simulink model "karamy"  (R2016b)
settings: Solver=ode23s  StartTime=0.0  StopTime=10  RelTol=.01
InitFcn:
  | init
values from neighbouring files (symbols this model uses):
  etta0 = x(3)    [KARAMY2.m]    (also in system10.mat = 0.574023203436; system20.mat = 0.293427975482; system30.mat = 0.568096136445)
  Ksm0 = x(1)    [KARAMY2.m]    (also in system10.mat = 0.523640532645; system20.mat = 0.612490346894; system30.mat = 0.775379405953)
settings Model: Creator=Mojtaba  LastModifiedBy=Mojtaba
settings SolverCC: ShapePreserveControl=EnableAll

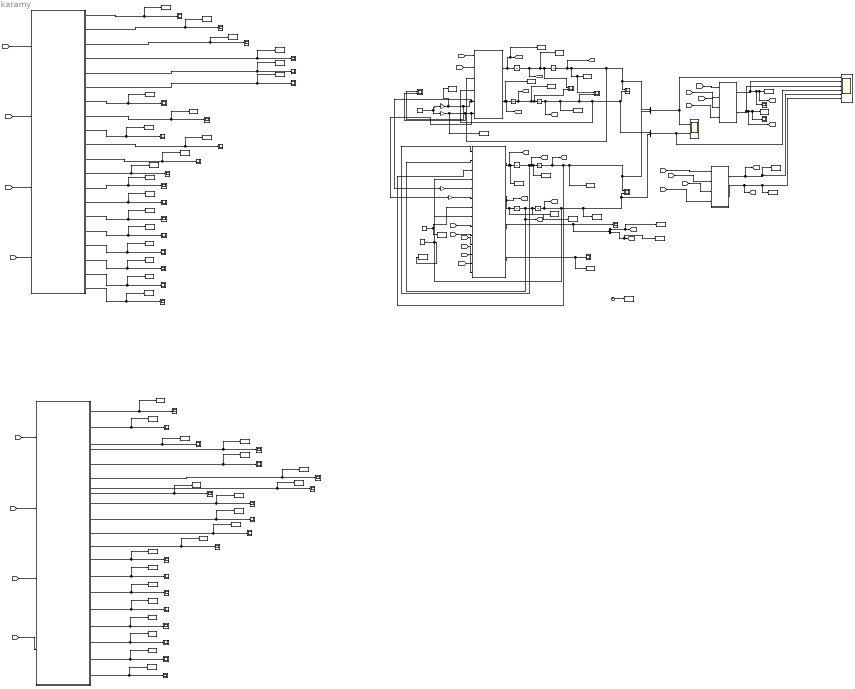
== system karamy ==
  Clock : Clock
  Constant : Constant  Value=Ksm0
  Constant1 : Constant  Value=etta0
  Demux : Demux  Outputs=2
  Dis : SignalGenerator  Amplitude=.1  Units=rad/sec
  Gain{,1..3} (4 alike) : Gain
  Integrator10 : Integrator  InitialCondition=.6
  Integrator11 : Integrator  InitialCondition=.1
  Integrator{8..9,12..13} (4 alike) : Integrator
  Integrator14 : Integrator  InitialCondition=.6
  Integrator15 : Integrator  InitialCondition=.1
  "Muscle1 " : MATLAB Function  TreatAsAtomicUnit=on
  Muscle2 : MATLAB Function  TreatAsAtomicUnit=on
  Mux5 : Mux  Inputs=2
  Mux6 : Mux  Inputs=2
  Subsystem10 : Subsystem
  Subsystem13 : Subsystem
  To Workspace : ToWorkspace  VariableName=u1  SampleTime=-1
  To Workspace1 : ToWorkspace  VariableName=ddqO2  SampleTime=-1
  To Workspace10 : ToWorkspace  VariableName=dqO1  SampleTime=-1
  To Workspace11 : ToWorkspace  VariableName=ddqO1  SampleTime=-1
  To Workspace12 : ToWorkspace  VariableName=qC1  SampleTime=-1
  To Workspace13 : ToWorkspace  VariableName=ddqC2  SampleTime=-1
  To Workspace14 : ToWorkspace  VariableName=ddxR2  SampleTime=-1
  To Workspace15 : ToWorkspace  VariableName=ddxL2  SampleTime=-1
  To Workspace16 : ToWorkspace  VariableName=ddxR1  SampleTime=-1
  To Workspace17 : ToWorkspace  VariableName=Ksm  SampleTime=-1
  To Workspace18 : ToWorkspace  VariableName=dis1  SampleTime=-1
  To Workspace19 : ToWorkspace  VariableName=dqO2  SampleTime=-1
  To Workspace2 : ToWorkspace  VariableName=time  SampleTime=-1
  To Workspace20 : ToWorkspace  VariableName=qO2  SampleTime=-1
  To Workspace21 : ToWorkspace  VariableName=dqC2  SampleTime=-1
  To Workspace22 : ToWorkspace  VariableName=ddxL1  SampleTime=-1
  To Workspace25 : ToWorkspace  VariableName=u2  SampleTime=-1
  To Workspace26 : ToWorkspace  VariableName=qO1  SampleTime=-1
  To Workspace27 : ToWorkspace  VariableName=dqC1  SampleTime=-1
  To Workspace28 : ToWorkspace  VariableName=qC2  SampleTime=-1
  To Workspace29 : ToWorkspace  VariableName=ddqC1  SampleTime=-1
  To Workspace3 : ToWorkspace  VariableName=dis2  SampleTime=-1
  To Workspace34 : ToWorkspace  VariableName=xR1  SampleTime=-1
  To Workspace35 : ToWorkspace  VariableName=xL1  SampleTime=-1
  To Workspace36 : ToWorkspace  VariableName=dxR1  SampleTime=-1
  To Workspace37 : ToWorkspace  VariableName=dxL1  SampleTime=-1
  To Workspace38 : ToWorkspace  VariableName=PR1  SampleTime=-1
  To Workspace39 : ToWorkspace  VariableName=PL1  SampleTime=-1
  To Workspace4 : ToWorkspace  VariableName=e2  SampleTime=-1
  To Workspace40 : ToWorkspace  VariableName=RRd1  SampleTime=-1
  To Workspace41 : ToWorkspace  VariableName=RRi1  SampleTime=-1
  To Workspace42 : ToWorkspace  VariableName=RLi1  SampleTime=-1
  To Workspace43 : ToWorkspace  VariableName=KpR1  SampleTime=-1
  To Workspace44 : ToWorkspace  VariableName=KpL1  SampleTime=-1
  To Workspace45 : ToWorkspace  VariableName=BpiL1  SampleTime=-1
  To Workspace46 : ToWorkspace  VariableName=BpdL1  SampleTime=-1
  To Workspace47 : ToWorkspace  VariableName=BpiR1  SampleTime=-1
  To Workspace48 : ToWorkspace  VariableName=BpdR1  SampleTime=-1
  To Workspace49 : ToWorkspace  VariableName=FR1  SampleTime=-1
  To Workspace5 : ToWorkspace  VariableName=de2  SampleTime=-1
  To Workspace50 : ToWorkspace  VariableName=FL1  SampleTime=-1
  To Workspace51 : ToWorkspace  VariableName=xR2  SampleTime=-1
  To Workspace52 : ToWorkspace  VariableName=xL2  SampleTime=-1
  To Workspace53 : ToWorkspace  VariableName=dxR2  SampleTime=-1
  To Workspace54 : ToWorkspace  VariableName=dxL2  SampleTime=-1
  To Workspace55 : ToWorkspace  VariableName=PR2  SampleTime=-1
  To Workspace56 : ToWorkspace  VariableName=PL2  SampleTime=-1
  To Workspace57 : ToWorkspace  VariableName=RRd2  SampleTime=-1
  To Workspace58 : ToWorkspace  VariableName=RRi2  SampleTime=-1
  To Workspace59 : ToWorkspace  VariableName=RLi2  SampleTime=-1
  To Workspace6 : ToWorkspace  VariableName=e1  SampleTime=-1
  To Workspace60 : ToWorkspace  VariableName=KpR2  SampleTime=-1
  To Workspace61 : ToWorkspace  VariableName=KpL2  SampleTime=-1
  To Workspace62 : ToWorkspace  VariableName=BpiL2  SampleTime=-1
  To Workspace63 : ToWorkspace  VariableName=BpdL2  SampleTime=-1
  To Workspace64 : ToWorkspace  VariableName=BpiR2  SampleTime=-1
  To Workspace65 : ToWorkspace  VariableName=BpdR2  SampleTime=-1
  To Workspace66 : ToWorkspace  VariableName=FR2  SampleTime=-1
  To Workspace67 : ToWorkspace  VariableName=FL2  SampleTime=-1
  To Workspace68 : ToWorkspace  VariableName=RLd1  SampleTime=-1
  To Workspace69 : ToWorkspace  VariableName=RLd2  SampleTime=-1
  To Workspace7 : ToWorkspace  VariableName=de1  SampleTime=-1
  To Workspace8 : ToWorkspace  VariableName=etta  SampleTime=-1
  To Workspace9 : ToWorkspace  VariableName=S  SampleTime=-1
  close loop 1 : MATLAB Function  TreatAsAtomicUnit=on
  comparison1 : Scope  NumInputPorts=6
  de1 : Scope
  e1 : Scope
  open  loop1 : MATLAB Function  TreatAsAtomicUnit=on
  q{1..5} (5 alike) : Scope  NumInputPorts=2
  teta1 : Scope  NumInputPorts=2
  u{,1..41} (42 alike) : Scope
  wires:
  open  loop1/1(ddq1) -> To Workspace11/1, [ddqO1], Integrator8/1
  open  loop1/2(ddq2) -> To Workspace1/1, [ddqO2], Integrator9/1
  Integrator9/1 -> [dqO2], To Workspace19/1, q5/2, Integrator11/1
  Integrator8/1 -> [dqO1], To Workspace10/1, q5/1, Integrator10/1
  Integrator13/1 -> To Workspace21/1, Integrator15/1, close loop 1/2(dq2), [dqC2]
  Integrator12/1 -> close loop 1/1(dq1), To Workspace27/1, Integrator14/1, [dqC1]
  Integrator15/1 -> [qC2], To Workspace28/1, Mux6/2, q3/2, close loop 1/4(q2)
  close loop 1/3(u) -> Demux/1, u/1
  Gain1/1 -> To Workspace3/1, q1/2, Gain3/1, open  loop1/6(dis2)
  Gain/1 -> To Workspace18/1, q1/1, Gain2/1, open  loop1/5(dis1)
  [dqC1] -> Subsystem10/4(dqC)
  [dqO1] -> Subsystem10/3(dqO)
  [qC1] -> Subsystem10/2(qC)
  [qO1] -> Subsystem10/1(qO)
  [dqC2] -> Subsystem13/4(dqC)
  [dqO2] -> Subsystem13/3(dqO)
  [qC2] -> Subsystem13/2(qC)
  [qO2] -> Subsystem13/1(qO)
  Constant/1 -> close loop 1/7(Ksm0), To Workspace17/1
  Constant1/1 -> close loop 1/8(etta0), To Workspace8/1
  Dis/1 -> Gain/1, Gain1/1
  Subsystem10/1(e) -> e1/1, [e1], To Workspace6/1, comparison1/2
  Subsystem10/2(de) -> comparison1/3, [de1], de1/1, To Workspace7/1
  Subsystem13/1(e) -> To Workspace4/1, comparison1/5, [e2]
  Subsystem13/2(de) -> [de2], To Workspace5/1, comparison1/6
  Integrator10/1 -> [qO1], q4/1, To Workspace26/1, Mux5/1, q2/1, open  loop1/3(q1)
  Mux5/1 -> teta1/1, comparison1/1
  Integrator11/1 -> [qO2], To Workspace20/1, q4/2, q2/2, Mux6/1, open  loop1/4(q2)
  Mux6/1 -> teta1/2, comparison1/4
  [dqO2] -> open  loop1/2(dq2)
  [dqO1] -> open  loop1/1(dq1)
  [qC1] -> "Muscle1 "/1(q)
  [dqC1] -> "Muscle1 "/2(dq)
  [u1] -> "Muscle1 "/4(deltaP)
  Demux/1 -> To Workspace/1, [u1]
  Demux/2 -> To Workspace25/1, [u2]
  "Muscle1 "/1(xR) -> To Workspace34/1, u1/1
  "Muscle1 "/2(xL) -> u2/1, To Workspace35/1
  "Muscle1 "/3(dxR) -> To Workspace36/1, u3/1
  "Muscle1 "/4(dxL) -> u4/1, To Workspace37/1
  "Muscle1 "/7(PR) -> To Workspace38/1, u5/1
  "Muscle1 "/8(PL) -> u6/1, To Workspace39/1
  "Muscle1 "/9(RRd) -> To Workspace40/1, u7/1
  "Muscle1 "/11(RRi) -> u8/1, To Workspace41/1
  "Muscle1 "/12(RLi) -> To Workspace42/1, u9/1
  "Muscle1 "/13(KpR) -> u10/1, To Workspace43/1
  "Muscle1 "/14(KpL) -> To Workspace44/1, u11/1
  "Muscle1 "/15(BpiL) -> u12/1, To Workspace45/1
  "Muscle1 "/16(BpdL) -> To Workspace46/1, u13/1
  "Muscle1 "/17(BpiR) -> u14/1, To Workspace47/1
  "Muscle1 "/18(BpdR) -> To Workspace48/1, u15/1
  "Muscle1 "/19(FR) -> u16/1, To Workspace49/1
  "Muscle1 "/20(FL) -> To Workspace50/1, u17/1
  [qC2] -> Muscle2/1(q)
  [dqC2] -> Muscle2/2(dq)
  [u2] -> Muscle2/4(deltaP)
  Muscle2/1(xR) -> u18/1, To Workspace51/1
  Muscle2/2(xL) -> To Workspace52/1, u27/1
  Muscle2/3(dxR) -> u28/1, To Workspace53/1
  Muscle2/4(dxL) -> To Workspace54/1, u29/1
  Muscle2/7(PR) -> u30/1, To Workspace55/1
  Muscle2/8(PL) -> To Workspace56/1, u31/1
  Muscle2/9(RRd) -> u32/1, To Workspace57/1
  Muscle2/11(RRi) -> To Workspace58/1, u33/1
  Muscle2/12(RLi) -> u34/1, To Workspace59/1
  Muscle2/13(KpR) -> To Workspace60/1, u19/1
  Muscle2/14(KpL) -> u20/1, To Workspace61/1
  Muscle2/15(BpiL) -> To Workspace62/1, u21/1
  Muscle2/16(BpdL) -> u22/1, To Workspace63/1
  Muscle2/17(BpiR) -> To Workspace64/1, u23/1
  Muscle2/18(BpdR) -> u24/1, To Workspace65/1
  Muscle2/19(FR) -> To Workspace66/1, u25/1
  Muscle2/20(FL) -> u26/1, To Workspace67/1
  "Muscle1 "/10(RLd) -> To Workspace68/1, u35/1
  Muscle2/10(RLd) -> To Workspace69/1, u36/1
  close loop 1/2(ddqC2) -> [ddqC2], To Workspace13/1, Integrator13/1
  Integrator14/1 -> [qC1], To Workspace12/1, Mux5/2, q3/1, close loop 1/3(q1)
  close loop 1/1(ddqC1) -> [ddqC1], To Workspace29/1, Integrator12/1
  Clock/1 -> To Workspace2/1
  close loop 1/4(S) -> To Workspace9/1, u37/1
  [ddqC1] -> "Muscle1 "/3(ddq)
  [ddqC2] -> Muscle2/3(ddq)
  Muscle2/5(ddxR) -> u38/1, To Workspace14/1
  Muscle2/6(ddxL) -> To Workspace15/1, u39/1
  "Muscle1 "/5(ddxR) -> To Workspace16/1, u40/1
  "Muscle1 "/6(ddxL) -> u41/1, To Workspace22/1
  Gain2/1 -> close loop 1/5(dis1)
  Gain3/1 -> close loop 1/6(dis2)
  [e1] -> close loop 1/9(e1)
  [e2] -> close loop 1/10(e2)
  [de2] -> close loop 1/12(de2)
  [de1] -> close loop 1/11(de1)
  [ddqO1] -> close loop 1/14(ddqO2)
  [ddqO2] -> close loop 1/13(ddqO1)

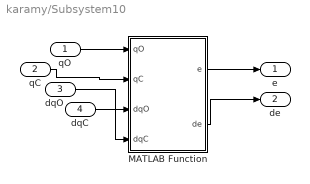
== system karamy/Subsystem10 ==
  qO : Inport
  qC : Inport  Port=2
  dqO : Inport  Port=3
  dqC : Inport  Port=4
  MATLAB Function : MATLAB Function  TreatAsAtomicUnit=on
  e : Outport
  de : Outport  Port=2
  wires:
  qO/1 -> MATLAB Function/1(qO)
  MATLAB Function/1(e) -> e/1
  dqC/1 -> MATLAB Function/4(dqC)
  dqO/1 -> MATLAB Function/3(dqO)
  qC/1 -> MATLAB Function/2(qC)
  MATLAB Function/2(de) -> de/1

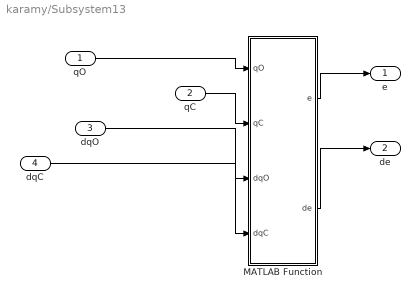
== system karamy/Subsystem13 ==
  qO : Inport
  qC : Inport  Port=2
  dqO : Inport  Port=3
  dqC : Inport  Port=4
  MATLAB Function : MATLAB Function  TreatAsAtomicUnit=on
  e : Outport
  de : Outport  Port=2
  wires:
  MATLAB Function/2(de) -> de/1
  qC/1 -> MATLAB Function/2(qC)
  dqO/1 -> MATLAB Function/3(dqO)
  dqC/1 -> MATLAB Function/4(dqC)
  MATLAB Function/1(e) -> e/1
  qO/1 -> MATLAB Function/1(qO)

== matlab function karamy/Muscle2 ==
  data: q input; dq input; ddq input; deltaP input; xR output; xL output; dxR output; dxL output; ddxR output; ddxL output; PR output; PL output; RRd output; RLd output; RRi output; RLi output; KpR output; KpL output; BpiL output; BpdL output; BpiR output; BpdR output; FR output; FL output
function [xR,xL,dxR,dxL,ddxR,ddxL,PR,PL,RRd,RLd,RRi,RLi,KpR,KpL,BpiL,BpdL,BpiR,BpdR,FR,FL] =Muscle2(q,dq,ddq,deltaP)
%% 1
n=3;
r=0.06; 
B_Li=.1;
B_Ld=.1;
B_Ri=.1;
B_Rd=.1;
%
B_0Li=.1;
B_0Ld=.1;
B_0Ri=.1;
B_0Rd=.1;
%
K_L=5;
K_R=5;
K_0L=5;
K_0R=5;
%
P_0R=1;  %420e3
P_0L=1;  %405e3
F_R=1;
F_L=1;
%% x dx  
xR=(pi+q)*r;
xL=(pi-q)*r;
dxR=(dq)*r;
dxL=(dq)*r;
ddxR=(ddq)*r; 
ddxL=(ddq)*r;
%% Pr  PL   
PR=P_0R+deltaP;
PL=P_0L+deltaP;
%% RRd  RLd   
RRd=n*(F_R-B_Rd*dxR-K_R*dxR);
RLd=n*(F_L-B_Ld*dxR-K_L*dxR);
%% RRi  RLi    
RRi=n*(F_R-B_Ri*dxR-K_R*dxR);
RLi=n*(F_L-B_Li*dxR-K_L*dxR);
%%  K        
KpR=K_0R+K_R*deltaP;
KpL=K_0L+K_L*deltaP;
%% B    
% left
BpiL=B_0Li+B_Li*deltaP;
BpdL=B_0Ld+B_Ld*deltaP;
% right
BpiR=B_0Ri+B_Ri*deltaP;
BpdR=B_0Rd+B_Rd*deltaP;
%% F 
FR=P_0R+F_R*deltaP;
FL=P_0L+F_L*deltaP;
end

== matlab function karamy/Muscle1  ==
  data: q input; dq input; ddq input; deltaP input; xR output; xL output; dxR output; dxL output; ddxR output; ddxL output; PR output; PL output; RRd output; RLd output; RRi output; RLi output; KpR output; KpL output; BpiL output; BpdL output; BpiR output; BpdR output; FR output; FL output
function [xR,xL,dxR,dxL,ddxR,ddxL,PR,PL,RRd,RLd,RRi,RLi,KpR,KpL,BpiL,BpdL,BpiR,BpdR,FR,FL] =Muscle1(q,dq,ddq,deltaP)
%% 1 B_Li 
r=0.07; 
n=6; %n2=3;
B_Li=.1;
B_Ld=.1;
B_Ri=.1;
B_Rd=.1;
%
B_0Li=.1;
B_0Ld=.1;
B_0Ri=.1;
B_0Rd=.1;
%
K_L=5;
K_R=5;
K_0L=5;
K_0R=5;
%
P_0R=1;  %420e3
P_0L=1;  %405e3
F_R=1;
F_L=1;
%% x dx  
xR=(pi+q)*r;
xL=(pi-q)*r;
dxR=(dq)*r;
dxL=(dq)*r;
ddxR=(ddq)*r; 
ddxL=(ddq)*r;
%% Pr  PL   
PR=P_0R+deltaP;
PL=P_0L+deltaP;
%% RRd  RLd   
RRd=n*(F_R-B_Rd*dxR-K_R*dxR);
RLd=n*(F_L-B_Ld*dxR-K_L*dxR);
%% RRi  RLi    
RRi=n*(F_R-B_Ri*dxR-K_R*dxR);
RLi=n*(F_L-B_Li*dxR-K_L*dxR);
%%  K        
KpR=K_0R+K_R*deltaP;
KpL=K_0L+K_L*deltaP;
%% B    
% left
BpiL=B_0Li+B_Li*deltaP;
BpdL=B_0Ld+B_Ld*deltaP;
% right
BpiR=B_0Ri+B_Ri*deltaP;
BpdR=B_0Rd+B_Rd*deltaP;
%% F 
FR=P_0R+F_R*deltaP;
FL=P_0L+F_L*deltaP;
end

== matlab function karamy/Subsystem10/MATLAB Function ==
  data: qO input; e output; qC input; dqO input; dqC input; de output
function [e,de]= fcn(qO,qC,dqO,dqC)
e=abs(qC-qO);
de=abs(dqC-dqO);
end

== matlab function karamy/Subsystem13/MATLAB Function ==
  data: qO input; e output; qC input; dqO input; dqC input; de output
function [e,de]= fcn(qO,qC,dqO,dqC)
e=abs(qC-qO);
de=abs(dqC-dqO);
end

== matlab function karamy/close loop 1 ==
  data: ddqC1 output; dq1 input; dq2 input; q1 input; q2 input; dis1 input; dis2 input; Ksm0 input; etta0 input; ddqC2 output; u output; e1 input; e2 input; S output; de1 input; de2 input; ddqO1 input; ddqO2 input
function [ddqC1,ddqC2,u,S]=systems(dq1,dq2,q1,q2,dis1,dis2,Ksm0,etta0,e1,e2,de1,de2,ddqO1,ddqO2)
%% params
l1=0.75;
lc1=0.5;
l2=l1;
lc2=lc1;
m1=7.5;
m2=7;
r1=0.07; %0.07
r2=0.06;  %0.06
n1=6;
n2=3;
I1=(m1*l1*l1)/12;
I2=(m2*l2*l2)/12;
g0=10;
%%
% K1R=20.748;K1L=20.748;F1R=.5e6;F1L=.5e6;B0Li=0.01;B1Li=0.01;B0Rd=0.01;
% B1Rd=0.01;B0Ld=0.01;
% B1Ld=0.01;B0Ri=0.01;B1Ri=0.01;P0R=420e3;P0L=405e3;r=.01;K0R=20.748;K0L=20.748;
% F0R=.5e6;F0L=.5e6;

B_1L1i=.1; %0.01
B_1L1d=.1;
B_1R1i=.1;
B_1R1d=.1;
%
B_1L2i=.1;
B_1L2d=.1;
B_1R2i=.1;
B_1R2d=.1;
%
B_0L1i=.1;
B_0L1d=.1;
B_0R1i=.1;
B_0R1d=.1;
B_0L2i=.1;
B_0L2d=.1;
B_0R2i=.1;
B_0R2d=.1;

K_1L1=5;
K_1R1=5;

K_1L2=5;
K_1R2=5;

K_0L1=5;
K_0R1=5;

K_0L2=5;
K_0R2=5;

P_0R1=1;  %420e3
P_0L1=1;  %405e3
P_0L2=P_0L1;
P_0R2=P_0R1;

F_1R1=1;
F_1L1=1;
F_1R2=1;
F_1L2=1;
F_2R1=1;
F_2L1=1;
F_2R2=1;
F_2L2=1;
%% 
dq=[dq1;dq2];
q=[q1;q2];
dis=[dis1;dis2];
%% d
d11=m2*(2*l1*lc2*cos(q2)+lc2*lc2+l1*l1)+m1*lc1*lc1+I1+I2;
d12=m2*(lc2*lc2+l1*lc2*cos(q2))+I2;
d21=d12;
d22=m2*lc2*lc2+I2;
d=[d11,d12;d21,d22];
dm=d;
d=pinv(d);
%% bA
if dq1<0
    bA1=-n1*(B_1L1i+B_1R1d)*r1*r1;
elseif dq1==0
    bA1=0;
else 
    bA1=n1*(B_1L1d+B_1R1i)*r1*r1;  
end
%
if dq2<0
    bA2=-n2*(B_1L2i+B_1R2d)*r2*r2;
elseif dq2==0
    bA2=0;
else 
    bA2=n2*(B_1L2d+B_1R2i)*r2*r2;   
end
%% aB
aB1=n1*r1*r1*(K_1R1-K_1L1);
aB2=n2*r2*r2*(K_1R2-K_1L2);
%% ac
ac1=2*F_2R1*P_0R1-F_1R1+2*F_2L1*P_0L1-F_1L1+r1*K_1R1*pi+r1*K_1L1*pi;
ac1=n1*r1*ac1;
ac2=2*F_2R2*P_0R2-F_1R2+2*F_2L2*P_0L2-F_1L2+r2*K_1R2*pi+r2*K_1L2*pi;
ac2=n2*r2*ac2;
%% h
h1=bA1*dq1+aB1*q1+ac1;
h2=bA2*dq2+aB2*q2+ac2;
h=[h1,0;0,h2];
%% bD   
if dq1<0
    bD1=-n1*r1*r1*(B_0L1i+B_1L1i*P_0L1+B_0R1d-B_1R1d*P_0R1);
elseif dq1==0
    bD1=0;
else 
    bD1=-n1*r1*r1*(B_0L1d-B_1L1d*P_0L1+B_0R1i+B_1R1i*P_0R1);  
end
%
if dq2<0
    bD2=-n2*r2*r2*(B_0L2i+B_1L2i*P_0L2+B_0R2d-B_1R2d*P_0R2);
elseif dq1==0
    bD2=0;
else 
    bD2=-n2*r2*r2*(B_0L2d-B_1L2d*P_0L2+B_0R2i+B_1R2i*P_0R2);  
end
bD=[bD1,0;0,bD2];
%% aE
aE1=K_1L1*P_0L1+K_1R1*P_0R1+K_0L1+K_0R1;
aE1=-n1*r1*r1*aE1;
aE2=K_1L2*P_0L2+K_1R2*P_0R2+K_0L2+K_0R2;
aE2=-n2*r2*r2*aE2;
aE=[aE1,0;0,aE2];
%% c
c21=m2*l1*sin(q2)*dq1;
c22=0;
c11=-m2*l1*lc2*dq2*sin(q2);
c12=-m2*l1*lc2*(dq1+dq2)*sin(q2);
c=[c11,c12;c21,c22];
%% g
g1=-m1*g0*lc1*sin(q1)-m2*g0*(l1*sin(q1)+lc2*sin(q1+q2));
g2=-m2*g0*lc2*sin(q1+q2);
g=[g1;g2];
%%  aF
aF1=F_2R1*P_0R1*P_0R1-F_1R1*P_0R1-F_2L1*P_0L1*P_0L1+...
    F_1L1*P_0L1+r1*K_1R1*P_0R1*pi+r1*K_0R1*pi-...
    r1*K_1L1*P_0L1*pi-r1*K_0L1*pi;
aF1=-n1*r1*aF1;
aF2=F_2R2*P_0R2*P_0R2-F_1R2*P_0R2+F_2L2*P_0L2*P_0L2+...
    F_1L2*P_0L2+r2*K_1R2*P_0R2*pi+r2*K_0R2*pi-...
    r2*K_1L2*P_0L2*pi-r2*K_0L2*pi;
aF2=-n2*r2*aF2;
aF=[aF1;aF2];
%%
% nn=2;
% Ksm=(10^nn)*ones(2);
% etta=(10^1)*ones(2,1);
% Ksm=1000*ones(2);
Ksm=Ksm0;
% k22=0.1;
% Ksm=1.*[k11,.0001;.0001,k22]; Ksm0,etta0
% Ksm= Ksm0;
% etta=[3;2];
etta=etta0;   %5-10
% X1=[qO1;qO2];
% X2=[dqO1;dqO2];
% X3=[ddqO1;ddqO2];
% F=(C*X2+K*X1+G-Ksm*X2);
%% Nouri
% phi1=-d*h;phi2=-d*(bD+c);phi3=-d*aE;phi4=-d*aF-d*g;phi5=-d;
% F=abs((phi1+Ksm)*X2)+abs(phi3*X1)+abs(phi4+phi5*dis);
% F=pinv(phi1)*F;
% S=phi2*X2+phi3*X1+phi4+phi5*dis+Ksm*X1;
% u=-F.*sign(S)-etta.*sign(S);
%% Karami
phi1=-d*h;phi2=-d*(bD+c);phi3=-d*aE;phi4=-d*aF-d*g;phi5=-d;
ee1=[e1;e2];
ee2=[de1;de2];
ddy_d=[ddqO1;ddqO2];
f=abs(phi2*ee2+phi3*ee1+phi4+phi5*dis);
g1=(phi1);
F=abs(f)+abs(g1*dis)+abs(ddy_d);
% F=f+g1*dis+ddy_d
F=g1*F;
S=ee2+Ksm*ee1;
%%
% F=M*F;
% S=abs(Ksm-C*pinv(M))*X2-pinv(M)*X1-pinv(M)*G-pinv(M)*dis;
%% approach 1
% u=-F.*sign(S)-etta.*sign(S);
%% approach 2
delta=0.001;
S1=tan(S./delta);
u=(-F-etta).*S1;
%% 
ddq=-d*h*u-d*(bD+c)*dq-d*aE*q-d*aF-d*g-d*dis;
ddqC1=ddq(1);
ddqC2=ddq(2);
end

== matlab function karamy/open  loop1 ==
  data: ddq1 output; dq1 input; dq2 input; q1 input; q2 input; dis1 input; dis2 input; ddq2 output
function [ddq1,ddq2]=systems(dq1,dq2,q1,q2,dis1,dis2)
%% params
l1=0.75;
lc1=0.5;
l2=l1;
lc2=lc1;
m1=7.5;
m2=7;
r1=0.07; %0.07
r2=0.06;  %0.06
n1=6;
n2=3;
I1=(m1*l1*l1)/12;
I2=(m2*l2*l2)/12;
g0=10;
%%
% K1R=20.748;K1L=20.748;F1R=.5e6;F1L=.5e6;B0Li=0.01;B1Li=0.01;B0Rd=0.01;
% B1Rd=0.01;B0Ld=0.01;
% B1Ld=0.01;B0Ri=0.01;B1Ri=0.01;P0R=420e3;P0L=405e3;r=.01;K0R=20.748;K0L=20.748;
% F0R=.5e6;F0L=.5e6;

B_1L1i=.1; %0.01
B_1L1d=.1;
B_1R1i=.1;
B_1R1d=.1;
%
B_1L2i=.1;
B_1L2d=.1;
B_1R2i=.1;
B_1R2d=.1;
%
B_0L1i=.1;
B_0L1d=.1;
B_0R1i=.1;
B_0R1d=.1;
B_0L2i=.1;
B_0L2d=.1;
B_0R2i=.1;
B_0R2d=.1;

K_1L1=5;
K_1R1=5;

K_1L2=5;
K_1R2=5;

K_0L1=5;
K_0R1=5;

K_0L2=5;
K_0R2=5;

P_0R1=1;  %420e3
P_0L1=1;  %405e3
P_0L2=P_0L1;
P_0R2=P_0R1;

F_1R1=1;
F_1L1=1;
F_1R2=1;
F_1L2=1;
F_2R1=1;
F_2L1=1;
F_2R2=1;
F_2L2=1;
%% 
dq=[dq1;dq2];
q=[q1;q2];
dis=[dis1;dis2];
%% d
d11=m2*(2*l1*lc2*cos(q2)+lc2*lc2+l1*l1)+m1*lc1*lc1+I1+I2;
d12=m2*(lc2*lc2+l1*lc2*cos(q2))+I2;
d21=d12;
d22=m2*lc2*lc2+I2;
d=[d11,d12;d21,d22];
d=pinv(d);
%% bA
if dq1<0
    bA1=-n1*(B_1L1i+B_1R1d)*r1*r1;
elseif dq1==0
    bA1=0;
else 
    bA1=n1*(B_1L1d+B_1R1i)*r1*r1;  
end
%
if dq2<0
    bA2=-n2*(B_1L2i+B_1R2d)*r2*r2;
elseif dq2==0
    bA2=0;
else 
    bA2=n2*(B_1L2d+B_1R2i)*r2*r2;   
end
%% aB
aB1=n1*r1*r1*(K_1R1-K_1L1);
aB2=n2*r2*r2*(K_1R2-K_1L2);
%% ac
ac1=2*F_2R1*P_0R1-F_1R1+2*F_2L1*P_0L1-F_1L1+r1*K_1R1*pi+r1*K_1L1*pi;
ac1=n1*r1*ac1;
ac2=2*F_2R2*P_0R2-F_1R2+2*F_2L2*P_0L2-F_1L2+r2*K_1R2*pi+r2*K_1L2*pi;
ac2=n2*r2*ac2;
%% h
h1=bA1*dq1+aB1*q1+ac1;
h2=bA2*dq2+aB2*q2+ac2;
h=[h1,0;0,h2];
%% bD   
if dq1<0
    bD1=-n1*r1*r1*(B_0L1i+B_1L1i*P_0L1+B_0R1d-B_1R1d*P_0R1);
elseif dq1==0
    bD1=0;
else 
    bD1=-n1*r1*r1*(B_0L1d-B_1L1d*P_0L1+B_0R1i+B_1R1i*P_0R1);  
end
%
if dq2<0
    bD2=-n2*r2*r2*(B_0L2i+B_1L2i*P_0L2+B_0R2d-B_1R2d*P_0R2);
elseif dq1==0
    bD2=0;
else 
    bD2=-n2*r2*r2*(B_0L2d-B_1L2d*P_0L2+B_0R2i+B_1R2i*P_0R2);  
end
bD=[bD1,0;0,bD2];
%% aE
aE1=K_1L1*P_0L1+K_1R1*P_0R1+K_0L1+K_0R1;
aE1=-n1*r1*r1*aE1;
aE2=K_1L2*P_0L2+K_1R2*P_0R2+K_0L2+K_0R2;
aE2=-n2*r2*r2*aE2;
aE=[aE1,0;0,aE2];
%% c
c21=m2*l1*sin(q2)*dq1;
c22=0;
c11=-m2*l1*lc2*dq2*sin(q2);
c12=-m2*l1*lc2*(dq1+dq2)*sin(q2);
c=[c11,c12;c21,c22];
%% g
g1=-m1*g0*lc1*sin(q1)-m2*g0*(l1*sin(q1)+lc2*sin(q1+q2));
g2=-m2*g0*lc2*sin(q1+q2);
g=[g1;g2];
%%  aF
aF1=F_2R1*P_0R1*P_0R1-F_1R1*P_0R1-F_2L1*P_0L1*P_0L1+...
    F_1L1*P_0L1+r1*K_1R1*P_0R1*pi+r1*K_0R1*pi-...
    r1*K_1L1*P_0L1*pi-r1*K_0L1*pi;
aF1=-n1*r1*aF1;
aF2=F_2R2*P_0R2*P_0R2-F_1R2*P_0R2+F_2L2*P_0L2*P_0L2+...
    F_1L2*P_0L2+r2*K_1R2*P_0R2*pi+r2*K_0R2*pi-...
    r2*K_1L2*P_0L2*pi-r2*K_0L2*pi;
aF2=-n2*r2*aF2;
aF=[aF1;aF2];
%% 
ddq=-(bD+c)*dq-aE*q-aF-g-dis;
ddq=d*ddq;
ddq1=ddq(1);
ddq2=ddq(2);
end
